simulink model "parte2"  (R2021b)
settings: Solver=FixedStepDiscrete  StartTime=0.0  StopTime=6  FixedStep=.03  RelTol=1e-3  EnableMultiTasking=on
PostLoadFcn:
  | try,
  | codertarget.arduinobase.registry.setBaudRate(gcs,115200)
  | disp('baud rate set to 115200 for external mode hardware serial')
  | baudrate='set_to_115200'
  | catch
  | disp('baud rate setting not needed in this version')
  | end
values from neighbouring files (symbols this model uses):
  EncCov = 2*pi /1336    (= 0.00470298301436)    [parte2_script.m]
  h = 0.03    [parte2_script.m]
  Ki = 0.2712    [parte2_script.m]
  Kp = 0.0271    [parte2_script.m]
undefined symbols (not defined in the file or in its folder): DiscIntNeverNeededParam
libraries: MinSegLibrary_M2V5 x2, simulink x1
settings Model: SimulationMode=external  ExtModeTrigDuration=2  Creator=Alec  LastModifiedBy=Dylan
settings SolverCC: AlgebraicLoopSolver=TrustRegion
settings DataIOCC: LimitDataPoints=on  SaveFormat=Array  ReturnWorkspaceOutputs=off
settings OptimizationCC: EnhancedBackFolding=on  PassReuseOutputArgsAs=Individual arguments  ExpressionDepthLimit=2147483647  ZeroExternalMemoryAtStartup=off  ZeroInternalMemoryAtStartup=off  MaxStackSize=64  OptimizeBlockOrder=speed  DifferentSizesBufferReuse=on  OptimizationCustomize=off  EfficientTunableParamExpr=on
settings DebuggingCC: UnderspecifiedInitializationDetection=Classic  MergeDetectMultiDrivingBlocksExec=none  ParameterTunabilityLossMsg=error  StateNameClashWarn=warning  SFUnexpectedBacktrackingDiag=warning  SFNoUnconditionalDefaultTransitionDiag=warning  SFExecutionAtInitializationDiag=none  SFMachineParentedDataDiag=warning  ArithmeticOperatorsInVariantConditions=warning
settings HardwareCC: ProdBitPerInt=16  ProdBitPerPointer=16  ProdBitPerSizeT=16  ProdBitPerPtrDiffT=16  ProdLargestAtomicFloat=None  ProdWordSize=8  ProdHWDeviceType=Atmel->AVR
settings ModelReferenceCC: PropagateSignalLabelsOutOfModel=off
settings SFSimCC: SimUseLocalCustomCode=off  MATLABDynamicMemAlloc=off  CustomCodeUndefinedFunction=UseInterfaceOnly
settings RTWCC: Description=Embedded Coder  SystemTargetFile=ert.tlc  HardwareBoard=Arduino Mega 2560  TemplateMakefile=ert_default_tmf  RTWVerbose=off  RTWUseLocalCustomCode=off  Toolchain=Arduino AVR  BuildConfiguration=Faster Runs
settings CodeAppCC: ForceParamTrailComments=on  IgnoreCustomStorageClasses=off  OperatorAnnotations=on  SimulinkDataObjDesc=on  SFDataObjDesc=on  CustomSymbolStrType=$N$R$M  InsertBlockDesc=on  InternalIdentifier=Classic
settings ERTTargetCC: SupportContinuousTime=on  SupportVariableSizeSignals=on  ExtModeTransport=3  ExtModeStaticAlloc=on  ExtModeStaticAllocSize=2048  ExtModeMexFile=ext_xcp  ExtModeIntrfLevel=Level2 - Open
settings ConfigComp: CovMetricSettings=dw  CovSaveCumulativeToWorkspaceVar=on  CovSaveSingleToWorkspaceVar=on  CovExternalEMLEnable=off

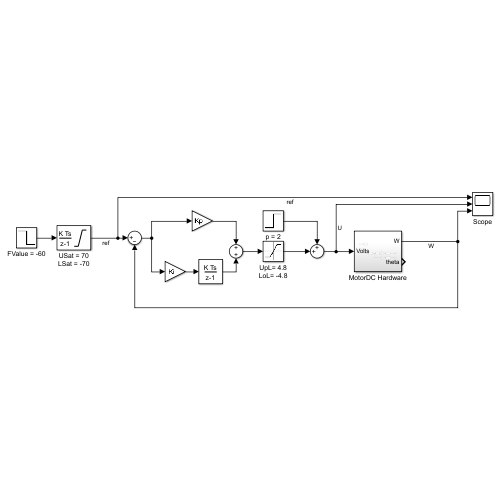
[thumbnail: Simulink's stored preview of the top-level diagram]
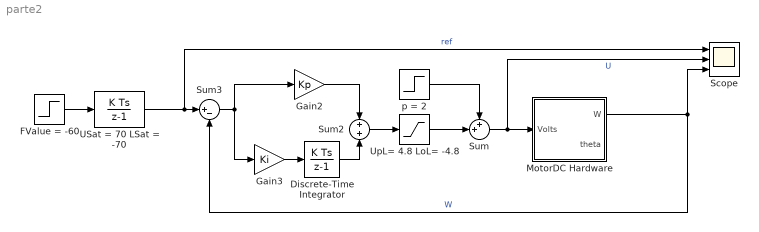
== system parte2 ==
  Discrete-Time Integrator : DiscreteIntegrator  SampleTime=h  ICPrevOutput=DiscIntNeverNeededParam  ICPrevScaledInput=DiscIntNeverNeededParam
  FValue = -60 : Step  After=-60  SampleTime=0
  Gain2 : Gain  Gain=Kp
  Gain3 : Gain  Gain=Ki
  MotorDC Hardware : Subsystem
  Scope : Scope  NumInputPorts=3
  Sum : Sum  Inputs=++|
  Sum2 : Sum  Inputs=+|+
  Sum3 : Sum  Inputs=|+-
  USat = 70 LSat = -70 : DiscreteIntegrator  SampleTime=h  LimitOutput=on  UpperSaturationLimit=70  LowerSaturationLimit=-70  ICPrevOutput=DiscIntNeverNeededParam  ICPrevScaledInput=DiscIntNeverNeededParam
  UpL= 4.8 LoL= -4.8 : Saturate  UpperLimit=4.8  LowerLimit=-4.8
  p = 2 : Step  Time=5  After=2  SampleTime=0
  wires:
  Sum3/1 -> Gain3/1, Gain2/1
  MotorDC Hardware/1(W) -> Sum3/2, Scope/3  "W"
  FValue = -60/1 -> USat = 70 LSat = -70/1
  Gain2/1 -> Sum2/1
  Gain3/1 -> Discrete-Time Integrator/1
  Sum2/1 -> UpL= 4.8 LoL= -4.8/1
  USat = 70 LSat = -70/1 -> Scope/1, Sum3/1  "ref"
  Discrete-Time Integrator/1 -> Sum2/2
  Sum/1 -> Scope/2, MotorDC Hardware/1(Volts)  "U"
  UpL= 4.8 LoL= -4.8/1 -> Sum/2
  p = 2/1 -> Sum/1

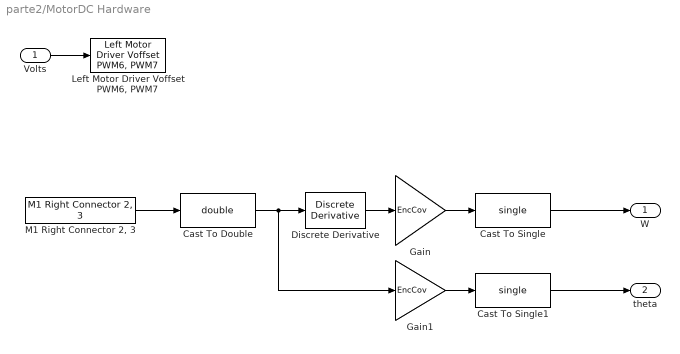
== system parte2/MotorDC Hardware ==
  Volts : Inport
  Cast To Double : DataTypeConversion  OutDataTypeStr=double
  Cast To Single : DataTypeConversion  OutDataTypeStr=single
  Cast To Single1 : DataTypeConversion  OutDataTypeStr=single
  Discrete Derivative : simulink/Discrete/Discrete Derivative  gainval=1.0  ICPrevScaledInput=0.0  OutMin=[]  OutMax=[]  OutDataType=fixdt(1, 16)  OutScaling=2^-10  DoSatur=off
  Gain : Gain  Gain=EncCov
  Gain1 : Gain  Gain=EncCov
  "Left Motor Driver Voffset PWM6, PWM7" : MinSegLibrary_M2V5/Left Motor Driver Voffset PWM6, PWM7  Vsupply=4.8  Voffset=0
      settings: SourceProductName=Rensselaer Arduino Support Package
  "M1 Right Connector 2, 3" : MinSegLibrary_M2V5/M1 Right Connector 2, 3  Encoder=0  PinA=2  PinB=3
      settings: SourceProductName=Rensselaer Arduino Support Package
  W : Outport
  theta : Outport  Port=2
  wires:
  Cast To Single/1 -> W/1
  Gain1/1 -> Cast To Single1/1
  Cast To Single1/1 -> theta/1
  "M1 Right Connector 2, 3"/1 -> Cast To Double/1
  Cast To Double/1 -> Gain1/1, Discrete Derivative/1
  Volts/1 -> "Left Motor Driver Voffset PWM6, PWM7"/1
  Discrete Derivative/1 -> Gain/1
  Gain/1 -> Cast To Single/1
